simulink model "Task3"  (R2022a)
settings: Solver=VariableStepAuto  StartTime=0.0  StopTime=20  RelTol=1e-3
settings Model: Creator=Family  LastModifiedBy=Family

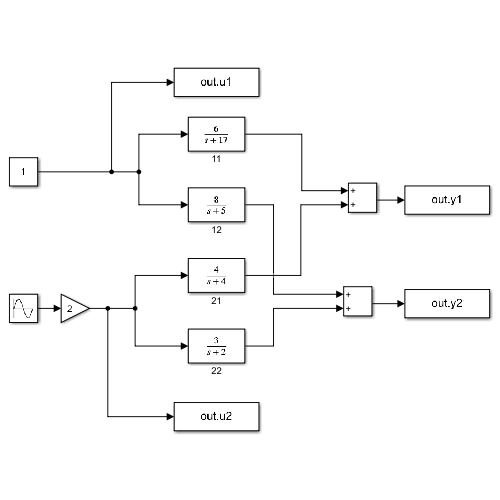
[thumbnail: Simulink's stored preview of the top-level diagram]
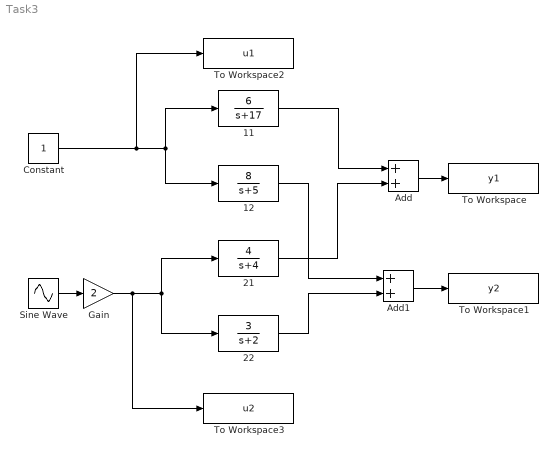
== system Task3 ==
  11 : TransferFcn  Numerator=[6]  Denominator=[1 17]
  12 : TransferFcn  Numerator=[8]  Denominator=[1 5]
  21 : TransferFcn  Numerator=[4]  Denominator=[1 4]
  22 : TransferFcn  Numerator=[3]  Denominator=[1 2]
  Add : Sum
  Add1 : Sum
  Constant : Constant  SampleTime=-1
  Gain : Gain  Gain=2
  Sine Wave : Sin  SampleTime=0
  To Workspace : ToWorkspace  VariableName=y1  SaveFormat=Timeseries  SampleTime=-1
  To Workspace1 : ToWorkspace  VariableName=y2  SaveFormat=Timeseries  SampleTime=-1
  To Workspace2 : ToWorkspace  VariableName=u1  SaveFormat=Timeseries  SampleTime=-1
  To Workspace3 : ToWorkspace  VariableName=u2  SaveFormat=Timeseries  SampleTime=-1
  wires:
  Add/1 -> To Workspace/1
  Sine Wave/1 -> Gain/1
  Gain/1 -> To Workspace3/1, 22/1, 21/1
  Constant/1 -> To Workspace2/1, 11/1, 12/1
  22/1 -> Add1/2
  12/1 -> Add1/1
  21/1 -> Add/2
  11/1 -> Add/1
  Add1/1 -> To Workspace1/1
